simulink model "diagramaTruxal"  (R2024b)
settings: Solver=VariableStepAuto  StartTime=0.0  StopTime=10.0  RelTol=1e-3
settings Model: Creator=estel  LastModifiedBy=estel

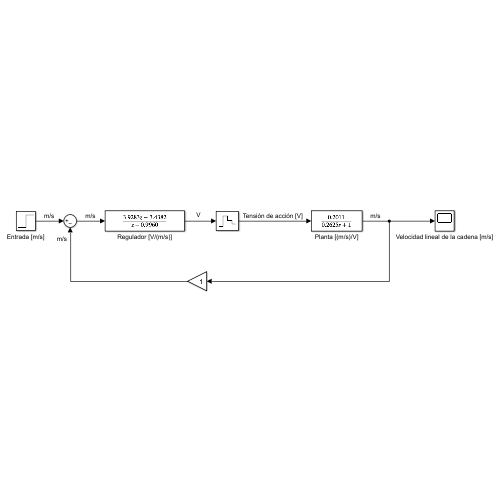
[thumbnail: Simulink's stored preview of the top-level diagram]
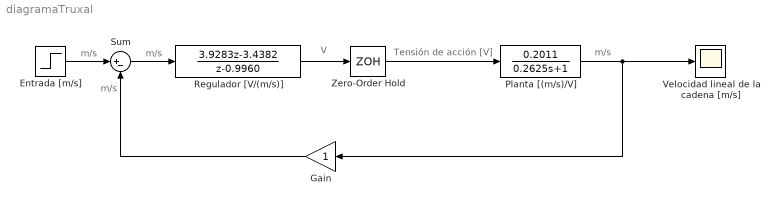
== system diagramaTruxal ==
  note: m/s
  note: m/s
  note: m/s
  note: m/s
  note: V
  note: Tensión de acción [V]
  Entrada [m/s] : Step  SampleTime=0
  Gain : Gain
  Planta [(m/s)/V] : TransferFcn  Numerator=[0.2011]  Denominator=[0.2625 1]
  Regulador [V/(m/s)] : DiscreteTransferFcn  Numerator=[3.9283 -3.4382]  Denominator=[1 -0.9960]
  Sum : Sum  Inputs=|+-
  Velocidad lineal de la cadena [m/s] : Scope
  Zero-Order Hold : ZeroOrderHold  SampleTime=-1
  wires:
  Entrada [m/s]/1 -> Sum/1
  Sum/1 -> Regulador [V/(m/s)]/1
  Regulador [V/(m/s)]/1 -> Zero-Order Hold/1
  Zero-Order Hold/1 -> Planta [(m/s)/V]/1
  Planta [(m/s)/V]/1 -> Gain/1, Velocidad lineal de la cadena [m/s]/1
  Gain/1 -> Sum/2
